simulink model "lazos_control_iqd0"  (R2020a)
settings: Solver=VariableStepAuto  StartTime=0.0  StopTime=10.0  RelTol=1e-3
model workspace: external: MATLAB File D:\Ferran\Facultad\UNCuyo\Meca\Automática y Máquinas Eléctricas\Proyecto final\matlab2\parametros_y_especs\parametros_y_especif.m (data not in the file)
undefined symbols (not defined in the file): R0, Rq, Rs
settings Model: Creator=Ferran  LastModifiedBy=Ferran

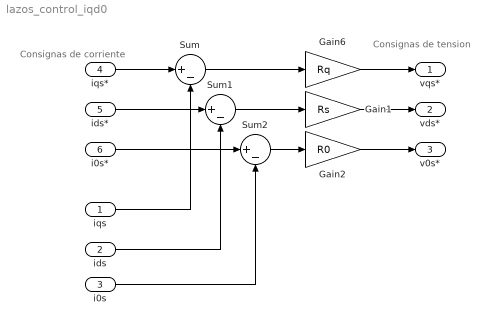
== system lazos_control_iqd0 ==
  note: Consignas
      | de
      | corriente
  note: Consignas de tension
  iqs : Inport
  ids : Inport  Port=2
  i0s : Inport  Port=3
  iqs* : Inport  Port=4
  ids* : Inport  Port=5
  i0s* : Inport  Port=6
  Gain1 : Gain  Gain=Rs
  Gain2 : Gain  Gain=R0
  Gain6 : Gain  Gain=Rq
  Sum : Sum  Inputs=|+-
  Sum1 : Sum  Inputs=|+-
  Sum2 : Sum  Inputs=|+-
  vqs* : Outport
  vds* : Outport  Port=2
  v0s* : Outport  Port=3
  wires:
  Gain6/1 -> vqs*/1
  Gain1/1 -> vds*/1
  Gain2/1 -> v0s*/1
  Sum/1 -> Gain6/1
  Sum1/1 -> Gain1/1
  iqs/1 -> Sum/2
  iqs*/1 -> Sum/1
  ids*/1 -> Sum1/1
  Sum2/1 -> Gain2/1
  i0s*/1 -> Sum2/1
  ids/1 -> Sum1/2
  i0s/1 -> Sum2/2
